simulink model "ES209A_CurrMeasCorrln"  (R2013b)
settings: Solver=FixedStepDiscrete  SolverMode=SingleTasking  StartTime=0.0  StopTime=1  FixedStep=0.000125  RelTol=1e-3
values from neighbouring files (symbols this model uses):
  CurrMeasCorrlnMaxErrCurr = DataDict.Calibration    [ES209A_CurrMeasCorrln_DataDict.m]
  CurrMeasCorrlnMaxStallCntr = DataDict.Calibration    [ES209A_CurrMeasCorrln_DataDict.m]
  CurrMeasCorrlnNtc0x04DFailStep = DataDict.Calibration    [ES209A_CurrMeasCorrln_DataDict.m]
  CurrMeasCorrlnNtc0x04DPassStep = DataDict.Calibration    [ES209A_CurrMeasCorrln_DataDict.m]
  CurrMeasCorrlnNtc0x04EFailStep = DataDict.Calibration    [ES209A_CurrMeasCorrln_DataDict.m]
  CurrMeasCorrlnNtc0x04EPassStep = DataDict.Calibration    [ES209A_CurrMeasCorrln_DataDict.m]
  ELECGLBPRM_IVTRCNT_CNT_U08 = DataDict.ConfigParam    [ES209A_CurrMeasCorrln_DataDict.m]
  FLTINJ_CURRMEASCORRLN_CURRMEASIDPTSIG = DataDict.Constant    [ES209A_CurrMeasCorrln_DataDict.m]
libraries: NxtrLim x2, simulink x1
(part 1 of 2)
settings Model: Creator=hzy4g9  LastModifiedBy=wzvp6q
settings SolverCC: AutoInsertRateTranBlk=on  InsertRTBMode=Always
settings DataIOCC: LimitDataPoints=off  SaveFormat=Structure  ReturnWorkspaceOutputs=on
settings OptimizationCC: BlockReduction=off  InlineParams=on  ZeroExternalMemoryAtStartup=off  ZeroInternalMemoryAtStartup=off  OptimizeModelRefInitCode=on  LifeSpan=1
settings DebuggingCC: SignalInfNanChecking=error  SignalRangeChecking=warning  UnderspecifiedInitializationDetection=Simplified  SolverPrmCheckMsg=error  InheritedTsInSrcMsg=error  DiscreteInheritContinuousMsg=error  SingleTaskRateTransMsg=error  TasksWithSamePriorityMsg=error  SigSpecEnsureSampleTimeMsg=error  CheckMatrixSingularityMsg=error  ParameterUnderflowMsg=error  ParameterPrecisionLossMsg=error  ParameterTunabilityLossMsg=error  FixptConstUnderflowMsg=warning  FixptConstOverflowMsg=warning  VectorMatrixConversionMsg=error  SignalLabelMismatchMsg=error  UnconnectedInputMsg=error  UnconnectedOutputMsg=error  UnconnectedLineMsg=error  SFcnCompatibilityMsg=error  UniqueDataStoreMsg=warning  BusObjectLabelMismatch=error  RootOutportRequireBusObject=error  AssertControl=DisableAll  ModelReferenceIOMsg=error  ModelReferenceVersionMismatchMessage=warning  ModelReferenceIOMismatchMessage=error  ModelReferenceCSMismatchMessage=warning  ModelReferenceDataLoggingMessage=error  StateNameClashWarn=warning  StrictBusMsg=ErrorOnBusTreatedAsVector  NonBusSignalsTreatedAsBus=error  SFUnexpectedBacktrackingDiag=error  SFInvalidInputDataAccessInChartInitDiag=error  SFNoUnconditionalDefaultTransitionDiag=error  SFTransitionOutsideNaturalParentDiag=error  SFUnconditionalTransitionShadowingDiag=error  SFUndirectedBroadcastEventsDiag=error
settings ModelReferenceCC: ModelReferenceNumInstancesAllowed=Single
settings RTWCC: SystemTargetFile=autosar.tlc  GenCodeOnly=on  TemplateMakefile=ert_default_tmf  Description=AUTOSAR  GenerateReport=on  ProcessScript=autosar_make_rtw_hook  LaunchReport=on
settings CodeAppCC: GenerateComments=off  IgnoreCustomStorageClasses=off  CustomSymbolStrType=$N$R$M  CustomSymbolStrBlkIO=$N$M  SimulinkBlockComments=off
settings STFCustomTargetCC: ParMdlRefBuildCompliant=on  CompOptLevelCompliant=on  IncludeMdlTerminateFcn=off  CombineOutputUpdateFcns=on  SuppressErrorStatus=on  ERTFirstTimeCompliant=on  ERTCustomFileBanners=on  SupportNonFinite=off  SupportComplex=off  SupportContinuousTime=off  SupportNonInlinedSFcns=off  MATLABClassNameForMDSCustomization=Simulink.SoftwareTarget.ERTCustomization  AutosarCompliant=on  GRTInterface=off  SystemTargetFile=autosar.tlc
settings ERTTargetCC: CodeReplacementLibrary=ANSI_C  ConcurrentExecutionCompliant=off  IncludeMdlTerminateFcn=off  SuppressErrorStatus=on  SupportNonFinite=off  SupportComplex=off  ModelStepFunctionPrototypeControlCompliant=off  CPPClassGenCompliant=off  AutosarCompliant=on  InlinedParameterPlacement=NonHierarchical  ERTCustomFileTemplate=example_file_process.tlc  EnableUserReplacementTypes=on

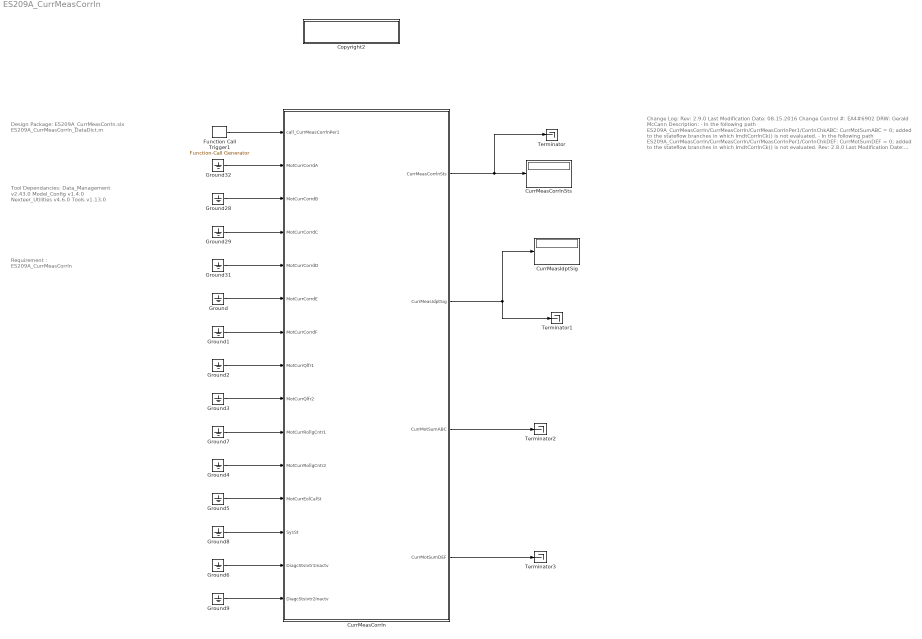
== system ES209A_CurrMeasCorrln ==
  note: Design Package:
      |
      | ES209A_CurrMeasCorrln.slx
      | ES209A_CurrMeasCorrln_DataDict.m
  note: Tool Dependancies:
      |
      | Data_Management v2.43.0
      | Model_Config v1.4.0
      | Nexteer_Utilities v4.6.0
      | Tools v1.13.0
  note: Requirement :
      |
      | ES209A_CurrMeasCorrln
  note: Change Log:
      |
      | Rev: 2.9.0
      | Last Modification Date: 08.15.2016
      | Change Control #: EA4#6902
      | DRW: Gerald McCann
      | Description:
      | - In the following path ES209A_CurrMeasCorrln/CurrMeasCorrln/CurrMeasCorrlnPer1/CorrlnChkABC:
      |    CurrMotSumABC = 0; added to the stateflow branches in which ImdtCorrlnCk() is not evaluated.
      | - In the following path ES209A_CurrMeasCorrln/CurrMeasCorrln/CurrMeasCorrlnPer1/CorrlnChkDEF:
      |    CurrMotSumDEF = 0; added to the stateflow branches in which ImdtCorrlnCk() is not evaluated.
      |
      | Rev: 2.8.0
      | Last Modification Date: 07.11.2016
      | Change Control #: EA4#6478
      | DRW: Gerald McCann
      | Description:
      | - In the following path, change the name of return value of ImdtCorrlnCk from CorrlnCk to ImdtCorrlnABC to match simulink block
      |    ES209A_CurrMeasCorrln/CurrMeasCorrln/CurrMeasCorrlnPer1/CorrlnChkABC
      | - In the following path, change the name of return value of ImdtCorrlnCk from CorrlnCk to ImdtCorrlnDEF to match simulink block
      |    ES209A_CurrMeasCorrln/CurrMeasCorrln/CurrMeasCorrlnPer1/CorrlnChkDEF
      | - In the following path, second condition [StallCntOutp >= kMaxStallCnt] changed to first condition.
      |    - ES209A_CurrMeasCorrln/CurrMeasCorrln/CurrMeasCorrlnPer1/Signal Availability/SigAvlChk1/SigAvlChkRev2
      | - Added return parameter CurrMotSum to ImdtCorrlnCk.  Source code unaffected as
      |    implementation already makes use of CurrMotSum.
      | - In stateflow CorrlnChkABC
      |    - Constant NTCNR_0X04D initial value changed to 77
      |    - Constant NTCNR_0X04D DataType changed to uint16
      | - In stateflow CorrlnChkDEF
      |    - Constant NTCNR_0X04E initial value changed to 78
      |    - Constant NTCNR_0X04E DataType changed to uint16
      | - Diagnostics warnings, Read Before Write, Write After Read and Write After Write has been
      |    changed to 'none' for the following blocks: NtcQlfr4D and NtcQlfr4E
      | - For simulation purposes only block ISO Fault Debounce Design stateflow has been modified
      |    to eliminate unconditional transitions
      | - Removed output port labels in the following paths due to signal label mismatch:
      |    - ES209A_CurrMeasCorrln/CurrMeasCorrln/CurrMeasCorrlnPer1/CorrlnChkABC/SetNtcSts/SetNtcSts/ISO Fault Debounce Design
      |    - ES209A_CurrMeasCorrln/CurrMeasCorrln/CurrMeasCorrlnPer1/CorrlnChkDEF/SetNtcSts/SetNtcSts/ISO Fault Debounce Design
      |
      | Rev: 2.7.0
      | Last Modification Date: 06.16.2016
      | Change Control #: EA4#6036
      | DRW: Raghavendran Mohan
      | Description:
      | - Added Fault Injection Mechanism for CurrMeasIdptSig
      |
      | Rev: 2.6.0
      | Last Modification Date: 04.22.2016
      | Change Control #: EA4#5281
      | DRW: Gerald McCann
      | Description:
      | - Signal Availability check is enabled only in enable/operate state.
      |
      | Rev: 2.5.0
      | Last Modification Date: 04.08.2016
      | Change Control #: EA4#5061
      | DRW: Praveen Devaraj(KPIT)
      | Description:
      | - Added two outputs CurrMotSumABC,CurrMotSumDEF and limiter added for these outputs.
      |
      | Rev: 2.4.0
      | Last Modification Date: 03.15.2016
      | Change Control #: Anomaly # EA4#2989     Comp   EA4#4533	     WCR # EA4#4747
      | DRW: N. Mahmud
      | Description:
      | - Fixed the datatype mismatch on CurrMeasCorrlnSts connection
      |
      | Rev: 2.3.0
      | Last Modification Date: 01.08.2016
      | Change Control #: EA4#2628	WCR # EA4#3283
      | DRW: N. Mahmud
      | Description:
      | - Requirement Linkage has been updated for the change described in the last version (Rev 2.2.0)
      |
      | Rev: 2.2.0
      | Last Modification Date: 12.07.2015
      | Change Control #: EA4#2628	WCR # EA4#2938
      | DRW: N. Mahmud
      | Description:
      | - Logic change in the number of independent signal  calculation for common mode failiure
      | - Change the kMaxStallCnt cal from 20 to 200 in the m file
      |
      | Rev: 2.1.0
      | Last Modification Date: 09.23.2015
      | Change Control #: WCR#1670
      | DRW: N. Mahmud
      | Description:
      | - Diagnostics has been disabled when gain/offset active: MotCurrEolCalSt is used to check that
      | - CurrMeasImdtCorrlnStsVldABC, CurrMeasLongTermCorrlnStsVldABC,
      |   CurrMeasImdtCorrlnStsVldDEF, CurrMeasLongTermCorrlnStsVldDEF are set to 1 as default.
      |
      | Rev: 1.0.0
      | Last Modification Date: 06.09.2015
      | Change Control #: ICR-
      | DRW: N. Mahmud
      | Description:
      | - Initial Release
      |
      | DRW: Nayeem Mahmud
      | Description:
      | ES209A Current Measurement Correlation
  Copyright2 : Subsystem  Description=|  mask(Copyright Information){none=on}
      | Copyright info block.                                               
      |                                                                     
      | Place copyright information at the top of every subsystem in design.
      mask prompts: none "No parameters"
      mask help: Place copyright information at the top of every subsystem in design.
      mask Display:
      | NxtrConf = 'Nexteer Confidential';
      | 
      | sys = bdroot; %handle for the current model ("system")
      | first = get_param(sys,'Created');
      | if(isempty(first))
      |     first = datestr(now,'yyyy');
      | else
      |     first = first(end-3:end);  %year is last four digits
      | end
      | 
      | last = get_param(sys,'LastModifiedDate');
      | if isempty(last)
      |     last = datestr(now,'yyyy');
      | else
      |     last = last(end-3:end);
      | end
      | 
      | if strcmp(first,last)
      |     fprintf('%s\nCopyright  %s Nexteer',NxtrConf,first);
      | else
      |     fprintf('%s\n%s%s-%s Nexteer',NxtrConf,char(169),first,last);
      | end
  CurrMeasCorrln : Subsystem  RequirementInfo={} %GIDa_ec0b3b79_5a07_49bd_97c9_8e172166434e
  CurrMeasCorrlnSts : Display
  CurrMeasIdptSig : Display
  Function Call Trigger1 : simulink/Ports & Subsystems/Function-Call Generator  RequirementInfo={} %GIDa_00b61420_5682_4f19_899b_6da543d44005  sample_time=0.000125  numberOfIterations=1
  Ground{,1..9,28..29,31..32} (14 alike) : Ground
  Terminator{,1..3} (4 alike) : Terminator
  wires:
  CurrMeasCorrln/1(CurrMeasCorrlnSts) -> Terminator/1, CurrMeasCorrlnSts/1
  CurrMeasCorrln/2(CurrMeasIdptSig) -> Terminator1/1, CurrMeasIdptSig/1
  Function Call Trigger1/1 -> CurrMeasCorrln/1(call_CurrMeasCorrlnPer1)
  Ground5/1 -> CurrMeasCorrln/12(MotCurrEolCalSt)
  Ground7/1 -> CurrMeasCorrln/10(MotCurrRollgCntr1)
  Ground28/1 -> CurrMeasCorrln/3(MotCurrCorrdB)
  Ground4/1 -> CurrMeasCorrln/11(MotCurrRollgCntr2)
  Ground9/1 -> CurrMeasCorrln/15(DiagcStsIvtr2Inactv)
  Ground6/1 -> CurrMeasCorrln/14(DiagcStsIvtr1Inactv)
  Ground31/1 -> CurrMeasCorrln/5(MotCurrCorrdD)
  Ground29/1 -> CurrMeasCorrln/4(MotCurrCorrdC)
  Ground2/1 -> CurrMeasCorrln/8(MotCurrQlfr1)
  Ground/1 -> CurrMeasCorrln/6(MotCurrCorrdE)
  Ground32/1 -> CurrMeasCorrln/2(MotCurrCorrdA)
  Ground8/1 -> CurrMeasCorrln/13(SysSt)
  Ground3/1 -> CurrMeasCorrln/9(MotCurrQlfr2)
  Ground1/1 -> CurrMeasCorrln/7(MotCurrCorrdF)
  CurrMeasCorrln/3(CurrMotSumABC) -> Terminator2/1
  CurrMeasCorrln/4(CurrMotSumDEF) -> Terminator3/1

== system ES209A_CurrMeasCorrln/Copyright2 ==

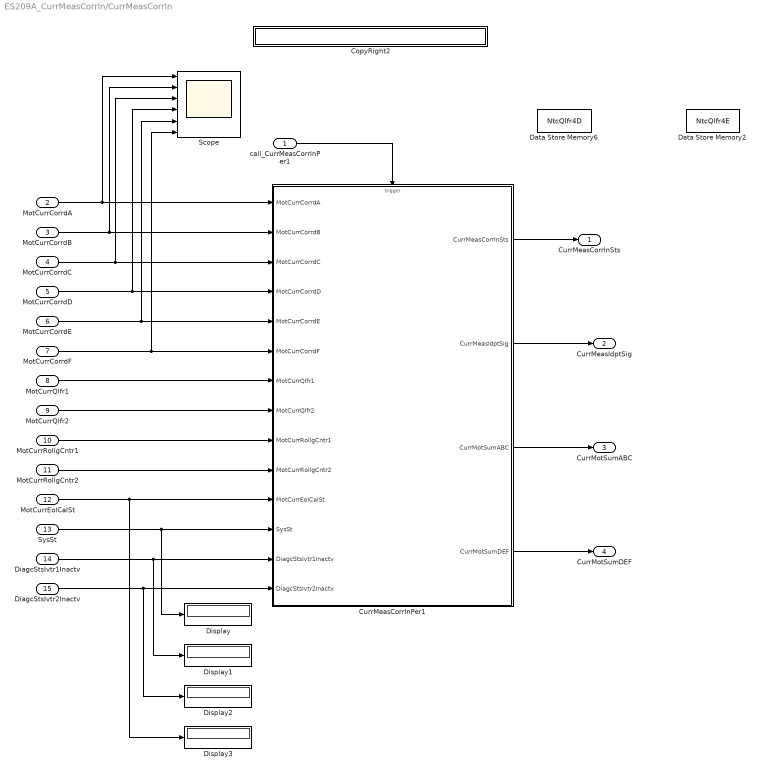
== system ES209A_CurrMeasCorrln/CurrMeasCorrln ==
  call_CurrMeasCorrlnPer1 : Inport
  MotCurrCorrdA : Inport  RequirementInfo={'linktype_rmi_doors' '0000c46e (/ESG Group/FDD Module Requirements/EA4 Specific/ES209A CurrMeasCorrln)' '#ES209A_104' 'true' 'REQ: ES209A_104' '' } %GIDa_0c74aa9f_9e88_4fad_92c6_c1c5b5def755  Port=2  OutDataTypeStr=single
  MotCurrCorrdB : Inport  RequirementInfo={'linktype_rmi_doors' '0000c46e (/ESG Group/FDD Module Requirements/EA4 Specific/ES209A CurrMeasCorrln)' '#ES209A_103' 'true' 'REQ: ES209A_103' '' } %GIDa_c4f83946_697c_4fbf_99fc_1a7b01ac928b  Port=3  OutDataTypeStr=single
  MotCurrCorrdC : Inport  RequirementInfo={'linktype_rmi_doors' '0000c46e (/ESG Group/FDD Module Requirements/EA4 Specific/ES209A CurrMeasCorrln)' '#ES209A_102' 'true' 'REQ: ES209A_102' '' } %GIDa_e8bdbe1c_0de3_460c_add6_42db4b0bf916  Port=4  OutDataTypeStr=single
  MotCurrCorrdD : Inport  RequirementInfo={'linktype_rmi_doors' '0000c46e (/ESG Group/FDD Module Requirements/EA4 Specific/ES209A CurrMeasCorrln)' '#ES209A_101' 'true' 'REQ: ES209A_101' '' } %GIDa_5fd63c82_c940_4205_a4b2_8a6f33b322f4  Port=5  OutDataTypeStr=single
  MotCurrCorrdE : Inport  RequirementInfo={'linktype_rmi_doors' '0000c46e (/ESG Group/FDD Module Requirements/EA4 Specific/ES209A CurrMeasCorrln)' '#ES209A_100' 'true' 'REQ: ES209A_100' '' } %GIDa_43c493df_4f0a_42bf_8466_dc5b3f8ce965  Port=6  OutDataTypeStr=single
  MotCurrCorrdF : Inport  RequirementInfo={'linktype_rmi_doors' '0000c46e (/ESG Group/FDD Module Requirements/EA4 Specific/ES209A CurrMeasCorrln)' '#ES209A_99' 'true' 'REQ: ES209A_99' '' } %GIDa_9f9bc708_ebce_4b8f_aa37_758e3dd2df64  Port=7  OutDataTypeStr=single
  MotCurrQlfr1 : Inport  RequirementInfo={'linktype_rmi_doors' '0000c46e (/ESG Group/FDD Module Requirements/EA4 Specific/ES209A CurrMeasCorrln)' '#ES209A_215' 'true' 'REQ: ES209A_215' '' } %GIDa_aa88c4e2_69a0_4fc7_a614_d2a8879a5609  Port=8
  MotCurrQlfr2 : Inport  RequirementInfo={'linktype_rmi_doors' '0000c46e (/ESG Group/FDD Module Requirements/EA4 Specific/ES209A CurrMeasCorrln)' '#ES209A_214' 'true' 'REQ: ES209A_214' '' } %GIDa_eed2eea5_fe21_4beb_a317_55bd282b43d2  Port=9
  MotCurrRollgCntr1 : Inport  RequirementInfo={'linktype_rmi_doors' '0000c46e (/ESG Group/FDD Module Requirements/EA4 Specific/ES209A CurrMeasCorrln)' '#ES209A_213' 'true' 'REQ: ES209A_213' '' } %GIDa_0df31c93_de9f_4bc8_bb2d_b19ad16d92b3  Port=10
  MotCurrRollgCntr2 : Inport  RequirementInfo={'linktype_rmi_doors' '0000c46e (/ESG Group/FDD Module Requirements/EA4 Specific/ES209A CurrMeasCorrln)' '#ES209A_212' 'true' 'REQ: ES209A_212' '' } %GIDa_a808d1c9_e453_4f42_bcf3_8307b2c8619b  Port=11
  MotCurrEolCalSt : Inport  RequirementInfo={} %GIDa_abcbe149_f782_4267_9a45_157caba417ed  Port=12
  SysSt : Inport  RequirementInfo={} %GIDa_8538c24b_5f6a_4d2a_9d09_038d40d09e05  Port=13  OutDataTypeStr=uint8
  DiagcStsIvtr1Inactv : Inport  RequirementInfo={} %GIDa_38774f0c_8ba6_46af_9c68_e8c1be2e73a7  Port=14  OutDataTypeStr=boolean
  DiagcStsIvtr2Inactv : Inport  RequirementInfo={} %GIDa_811cc2e1_8a27_4ac8_82c1_1322cbb91599  Port=15  OutDataTypeStr=boolean
  CopyRight2 : Subsystem  Description=|  mask(Copyright Information){none=on}
      | Copyright info block.                                               
      |                                                                     
      | Place copyright information at the top of every subsystem in design.
      mask prompts: none "No parameters"
      mask help: Place copyright information at the top of every subsystem in design.
      mask Display:
      | NxtrConf = 'Nexteer Confidential';
      | 
      | sys = bdroot; %handle for the current model ("system")
      | first = get_param(sys,'Created');
      | first = first(end-3:end);  %year is last four digits
      | 
      | last = get_param(sys,'LastModifiedDate');
      | if isempty(last)
      |     last = datestr(now,'yyyy');
      | else
      |     last = last(end-3:end);
      | end
      | 
      | if strcmp(first,last)
      |     fprintf('%s -- Copyright %s Nexteer',NxtrConf,first)
      | else
      |     fprintf('%s -- %s%s- %s Nexteer',NxtrConf,char(169),first,last)
      | end
  CurrMeasCorrlnPer1 : Subsystem  RequirementInfo={'linktype_rmi_doors' '0000c46e (/ESG Group/FDD Module Requirements/EA4 Specific/ES209A CurrMeasCorrln)' '#ES209A_262' 'true' 'REQ: ES209A_262' '' } %GIDa_55579703_5885_40a5_a6ff_7209441b4d74  TreatAsAtomicUnit=on
  Data Store Memory2 : DataStoreMemory  DataStoreName=NtcQlfr4E  OutDataTypeStr=uint8
      settings: AttributesFormatString=|
      | Simulation Purpose Only.
      | Do Not Code this block
      | Diagnostic Manager Owns this requirement
  Data Store Memory6 : DataStoreMemory  DataStoreName=NtcQlfr4D  OutDataTypeStr=uint8
      settings: AttributesFormatString=|
      | Simulation Purpose Only.
      | Do Not Code this block
      | Diagnostic Manager Owns this requirement
  Display{,1..3} (4 alike) : Display
  Scope : Scope  NumInputPorts=6
      settings: YMin=-30~-30~-5~-5~-5~-5  YMax=30~25~5~5~5~5  SaveName=ScopeData2
  CurrMeasCorrlnSts : Outport  RequirementInfo={'linktype_rmi_doors' '0000c46e (/ESG Group/FDD Module Requirements/EA4 Specific/ES209A CurrMeasCorrln)' '#ES209A_205' 'true' 'REQ: ES209A_205' '' } %GIDa_1cc70fdd_56e1_4fc7_8a0b_3b5472613135
  CurrMeasIdptSig : Outport  RequirementInfo={'linktype_rmi_doors' '0000c46e (/ESG Group/FDD Module Requirements/EA4 Specific/ES209A CurrMeasCorrln)' '#ES209A_216' 'true' 'REQ: ES209A_216' '' } %GIDa_d8a59612_7cd1_4e21_946e_1ecb99779eae  Port=2
  CurrMotSumABC : Outport  RequirementInfo={'linktype_rmi_doors' '0000c46e (/ESG Group/FDD Module Requirements/EA4 Specific/ES209A_CurrMeasCorrln)' '#ES209A_276' 'true' 'REQ: ES209A_276' '' } %GIDa_6a109cf6_d31d_4752_8888_2bcd8313dc3b  Port=3
  CurrMotSumDEF : Outport  RequirementInfo={'linktype_rmi_doors' '0000c46e (/ESG Group/FDD Module Requirements/EA4 Specific/ES209A_CurrMeasCorrln)' '#ES209A_277' 'true' 'REQ: ES209A_277' '' } %GIDa_ea0a91c7_9f07_4e8d_b88b_4e34ddd11616  Port=4
  wires:
  call_CurrMeasCorrlnPer1/1 -> CurrMeasCorrlnPer1/Trigger
  MotCurrCorrdC/1 -> Scope/3, CurrMeasCorrlnPer1/3(MotCurrCorrdC)
  MotCurrCorrdA/1 -> Scope/1, CurrMeasCorrlnPer1/1(MotCurrCorrdA)
  MotCurrCorrdD/1 -> Scope/4, CurrMeasCorrlnPer1/4(MotCurrCorrdD)
  MotCurrQlfr1/1 -> CurrMeasCorrlnPer1/7(MotCurrQlfr1)
  MotCurrCorrdF/1 -> Scope/6, CurrMeasCorrlnPer1/6(MotCurrCorrdF)
  MotCurrCorrdB/1 -> Scope/2, CurrMeasCorrlnPer1/2(MotCurrCorrdB)
  MotCurrQlfr2/1 -> CurrMeasCorrlnPer1/8(MotCurrQlfr2)
  MotCurrRollgCntr1/1 -> CurrMeasCorrlnPer1/9(MotCurrRollgCntr1)
  MotCurrRollgCntr2/1 -> CurrMeasCorrlnPer1/10(MotCurrRollgCntr2)
  MotCurrCorrdE/1 -> Scope/5, CurrMeasCorrlnPer1/5(MotCurrCorrdE)
  CurrMeasCorrlnPer1/1(CurrMeasCorrlnSts) -> CurrMeasCorrlnSts/1
  CurrMeasCorrlnPer1/2(CurrMeasIdptSig) -> CurrMeasIdptSig/1
  MotCurrEolCalSt/1 -> Display3/1, CurrMeasCorrlnPer1/11(MotCurrEolCalSt)
  SysSt/1 -> Display/1, CurrMeasCorrlnPer1/12(SysSt)
  DiagcStsIvtr1Inactv/1 -> Display1/1, CurrMeasCorrlnPer1/13(DiagcStsIvtr1Inactv)
  DiagcStsIvtr2Inactv/1 -> Display2/1, CurrMeasCorrlnPer1/14(DiagcStsIvtr2Inactv)
  CurrMeasCorrlnPer1/3(CurrMotSumABC) -> CurrMotSumABC/1
  CurrMeasCorrlnPer1/4(CurrMotSumDEF) -> CurrMotSumDEF/1

== system ES209A_CurrMeasCorrln/CurrMeasCorrln/CopyRight2 ==

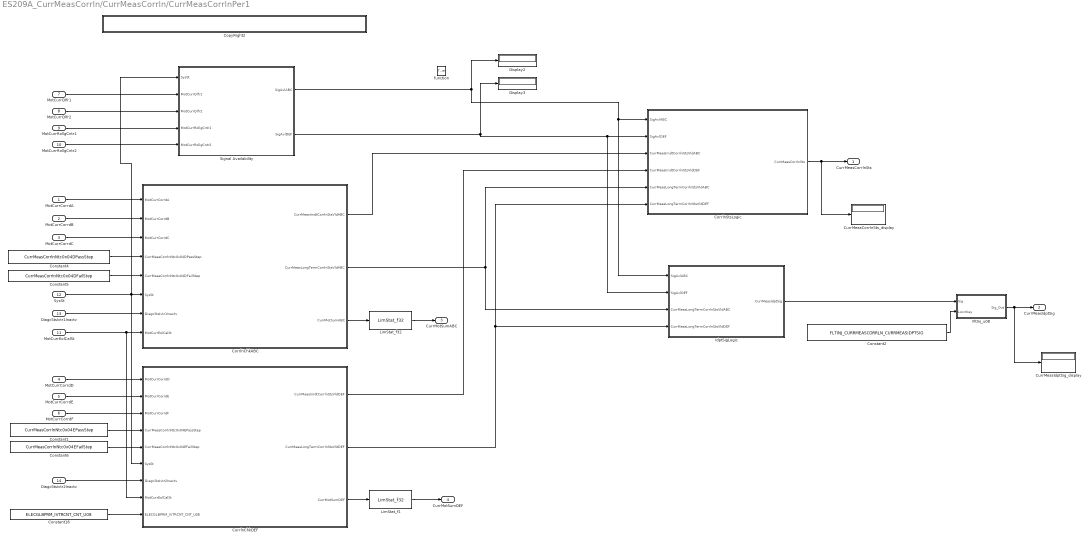
== system ES209A_CurrMeasCorrln/CurrMeasCorrln/CurrMeasCorrlnPer1 ==
  MotCurrCorrdA : Inport  RequirementInfo={} %GIDa_1b4be831_2b7f_4bad_8ca7_c41d6d58feee
  MotCurrCorrdB : Inport  RequirementInfo={} %GIDa_500faeb4_9506_45cf_9bc9_0622a43ff9e4  Port=2
  MotCurrCorrdC : Inport  RequirementInfo={} %GIDa_bdd58e2d_11b0_4592_a6cb_cf558d278bca  Port=3
  MotCurrCorrdD : Inport  RequirementInfo={} %GIDa_1787db15_a767_43f2_bc85_acb71f8d69c6  Port=4
  MotCurrCorrdE : Inport  RequirementInfo={} %GIDa_b914ba1e_8e7d_4f95_9ec4_a4f9530234f8  Port=5
  MotCurrCorrdF : Inport  RequirementInfo={} %GIDa_90fedd66_ffe2_4248_b2d7_fc88368a78d6  Port=6
  MotCurrQlfr1 : Inport  RequirementInfo={} %GIDa_549edda9_9c07_47e0_960b_2f7219c5afa3  Port=7
  MotCurrQlfr2 : Inport  RequirementInfo={} %GIDa_6f0dc6ab_4498_4871_aa7d_039a645c93f3  Port=8
  MotCurrRollgCntr1 : Inport  RequirementInfo={} %GIDa_941568a4_4b86_4eee_9c4b_01a9e8a0d271  Port=9
  MotCurrRollgCntr2 : Inport  RequirementInfo={} %GIDa_6bb84625_6e4a_46ad_a031_3a9a545a3e69  Port=10
  MotCurrEolCalSt : Inport  RequirementInfo={'linktype_rmi_doors' '0000c46e (/ESG Group/FDD Module Requirements/EA4 Specific/ES209A CurrMeasCorrln)' '#ES209A_263' 'true' 'REQ: ES209A_263' '' ; 'linktype_rmi_doors' '0000c46e (/ESG Group/FDD Module Requirements/EA4 Specific/ES209A CurrMeasCorrln)' '#ES209A_264' 'true' 'REQ: ES209A_264' '' ; 'linktype_rmi_doors' '0000c46e (/ESG Group/FDD Module Requirements/EA4 Specific/ES209A CurrMeasCorrln)' '#ES209A_263' 'true' 'REQ: ES209A_263' '' } %GIDa_c49b2222_d3c8_435a_aa49_2a5d2eee96f8  Port=11
  SysSt : Inport  RequirementInfo={'linktype_rmi_doors' '0000c46e (/ESG Group/FDD Module Requirements/EA4 Specific/ES209A CurrMeasCorrln)' '#ES209A_263' 'true' 'REQ: ES209A_263' '' ; 'linktype_rmi_doors' '0000c46e (/ESG Group/FDD Module Requirements/EA4 Specific/ES209A CurrMeasCorrln)' '#ES209A_264' 'true' 'REQ: ES209A_264' '' ; 'linktype_rmi_doors' '0000c46e (/ESG Group/FDD Module Requirements/EA4 Specific/ES209A CurrMeasCorrln)' '#ES209A_263' 'true' 'REQ: ES209A_263' '' } %GIDa_7eb989da_9939_43d3_b23d_4ca6ddd74654  Port=12  OutDataTypeStr=uint8
  DiagcStsIvtr1Inactv : Inport  RequirementInfo={'linktype_rmi_doors' '0000c46e (/ESG Group/FDD Module Requirements/EA4 Specific/ES209A CurrMeasCorrln)' '#ES209A_263' 'true' 'REQ: ES209A_263' '' ; 'linktype_rmi_doors' '0000c46e (/ESG Group/FDD Module Requirements/EA4 Specific/ES209A CurrMeasCorrln)' '#ES209A_263' 'true' 'REQ: ES209A_263' '' ; 'linktype_rmi_doors' '0000c46e (/ESG Group/FDD Module Requirements/EA4 Specific/ES209A CurrMeasCorrln)' '#ES209A_265' 'true' 'REQ: ES209A_265' '' } %GIDa_52cd4757_636a_4123_80e9_de329e501eb0  Port=13
  DiagcStsIvtr2Inactv : Inport  RequirementInfo={'linktype_rmi_doors' '0000c46e (/ESG Group/FDD Module Requirements/EA4 Specific/ES209A CurrMeasCorrln)' '#ES209A_264' 'true' 'REQ: ES209A_264' '' ; 'linktype_rmi_doors' '0000c46e (/ESG Group/FDD Module Requirements/EA4 Specific/ES209A CurrMeasCorrln)' '#ES209A_265' 'true' 'REQ: ES209A_265' '' } %GIDa_ae52e87f_c4e9_4b70_9292_5a6f0defc3c4  Port=14
  function : TriggerPort  TriggerType=function-call
  Constant1 : Constant  Value=CurrMeasCorrlnNtc0x04EPassStep
  Constant18 : Constant  RequirementInfo={'linktype_rmi_doors' '0000c46e (/ESG Group/FDD Module Requirements/EA4 Specific/ES209A CurrMeasCorrln)' '#ES209A_264' 'true' 'REQ: ES209A_264' '' } %GIDa_30da442b_a6bf_42bc_be81_91df8133d060  Value=ELECGLBPRM_IVTRCNT_CNT_U08
  Constant2 : Constant  Value=FLTINJ_CURRMEASCORRLN_CURRMEASIDPTSIG
  Constant4 : Constant  Value=CurrMeasCorrlnNtc0x04DPassStep
  Constant5 : Constant  Value=CurrMeasCorrlnNtc0x04DFailStep
  Constant6 : Constant  Value=CurrMeasCorrlnNtc0x04EFailStep
  CopyRight2 : Subsystem  Description=|  mask(Copyright Information){none=on}
      | Copyright info block.                                               
      |                                                                     
      | Place copyright information at the top of every subsystem in design.
      mask prompts: none "No parameters"
      mask help: Place copyright information at the top of every subsystem in design.
      mask Display:
      | NxtrConf = 'Nexteer Confidential';
      | 
      | sys = bdroot; %handle for the current model ("system")
      | first = get_param(sys,'Created');
      | first = first(end-3:end);  %year is last four digits
      | 
      | last = get_param(sys,'LastModifiedDate');
      | if isempty(last)
      |     last = datestr(now,'yyyy');
      | else
      |     last = last(end-3:end);
      | end
      | 
      | if strcmp(first,last)
      |     fprintf('%s -- Copyright %s Nexteer',NxtrConf,first)
      | else
      |     fprintf('%s -- %s%s- %s Nexteer',NxtrConf,char(169),first,last)
      | end
  CorrlnChkABC : Stateflow chart  TreatAsAtomicUnit=on
  CorrlnChkDEF : Stateflow chart  TreatAsAtomicUnit=on
  CorrlnStsLogic : Subsystem  RequirementInfo={} %GIDa_a00f341f_7944_4604_9319_bb050268a085
  CurrMeasCorrlnSts_display : Display
  CurrMeasIdptSig_display : Display
  Display2 : Display
  Display3 : Display
  FltInj_u08 : Subsystem  RequirementInfo={'linktype_rmi_doors' '0000c46e (/ESG Group/FDD Module Requirements/EA4 Specific/ES209A_CurrMeasCorrln)' '#ES209A_280' 'true' 'REQ: ES209A_280' '' } %GIDa_04468b6b_fc20_408a_acd8_ab774034357d  TreatAsAtomicUnit=on  VariantControl=FLTINJENA ~= STD_ON  mask(Fault_Injection){}
      mask help: Simulation mode is just a pass-thru.
  IdptSigLogic : Subsystem  RequirementInfo={} %GIDa_ea49a6a8_9dd9_4522_a425_2915623b798a
  LimStat_f1 : NxtrLim/LimStat_f32  LoLim=CurrMotSumDEF.EngMin  HiLim=CurrMotSumDEF.EngMax
      settings: AttributesFormatString=|
      | Low Limit: %<LoLim>
      | High Limit:%<HiLim>
  LimStat_f32 : NxtrLim/LimStat_f32  LoLim=CurrMotSumABC.EngMin  HiLim=CurrMotSumABC.EngMax
      settings: AttributesFormatString=|
      | Low Limit: %<LoLim>
      | High Limit:%<HiLim>
  Signal Availability : Subsystem  RequirementInfo={} %GIDa_b157c1ee_10a9_448e_9e7d_b9c83f2081ec
  CurrMeasCorrlnSts : Outport  RequirementInfo={} %GIDa_7d108d83_7d1e_4d9a_a3d7_d8c403dededd
  CurrMeasIdptSig : Outport  RequirementInfo={} %GIDa_f7dae694_b925_4279_806a_2573b5172d71  Port=2
  CurrMotSumABC : Outport  Port=3
  CurrMotSumDEF : Outport  Port=4
  wires:
  MotCurrCorrdB/1 -> CorrlnChkABC/2(MotCurrCorrdB)
  MotCurrCorrdA/1 -> CorrlnChkABC/1(MotCurrCorrdA)
  Signal Availability/2(SigAvlDEF) -> IdptSigLogic/2(SigAvlDEF), CorrlnStsLogic/2(SigAvlDEF), Display3/1
  MotCurrCorrdC/1 -> CorrlnChkABC/3(MotCurrCorrdC)
  CorrlnChkABC/2(CurrMeasLongTermCorrlnStsVldABC) -> IdptSigLogic/3(CurrMeasLongTermCorrlnStsVldABC), CorrlnStsLogic/5(CurrMeasLongTermCorrlnStsVldABC)
  Constant4/1 -> CorrlnChkABC/4(CurrMeasCorrlnNtc0x04DPassStep)
  Constant5/1 -> CorrlnChkABC/5(CurrMeasCorrlnNtc0x04DFailStep)
  Constant1/1 -> CorrlnChkDEF/4(CurrMeasCorrlnNtc0x04EPassStep)
  Constant6/1 -> CorrlnChkDEF/5(CurrMeasCorrlnNtc0x04EFailStep)
  MotCurrCorrdD/1 -> CorrlnChkDEF/1(MotCurrCorrdD)
  MotCurrCorrdE/1 -> CorrlnChkDEF/2(MotCurrCorrdE)
  MotCurrCorrdF/1 -> CorrlnChkDEF/3(MotCurrCorrdF)
  DiagcStsIvtr2Inactv/1 -> CorrlnChkDEF/7(DiagcStsIvtr2Inactv)
  Constant18/1 -> CorrlnChkDEF/9(ELECGLBPRM_IVTRCNT_CNT_U08)
  SysSt/1 -> CorrlnChkDEF/6(SysSt), Signal Availability/1(SysSt), CorrlnChkABC/6(SysSt)
  DiagcStsIvtr1Inactv/1 -> CorrlnChkABC/7(DiagcStsIvtr1Inactv)
  MotCurrEolCalSt/1 -> CorrlnChkDEF/8(MotCurrEolCalSt), CorrlnChkABC/8(MotCurrEolCalSt)
  IdptSigLogic/1(CurrMeasIdptSig) -> FltInj_u08/1(Sig)
  CorrlnStsLogic/1(CurrMeasCorrlnSts) -> CurrMeasCorrlnSts_display/1, CurrMeasCorrlnSts/1
  Signal Availability/1(SigAvlABC) -> IdptSigLogic/1(SigAvlABC), CorrlnStsLogic/1(SigAvlABC), Display2/1
  CorrlnChkABC/1(CurrMeasImdtCorrlnStsVldABC) -> CorrlnStsLogic/3(CurrMeasImdtCorrlnStsVldABC)
  CorrlnChkDEF/1(CurrMeasImdtCorrlnStsVldDEF) -> CorrlnStsLogic/4(CurrMeasImdtCorrlnStsVldDEF)
  CorrlnChkDEF/2(CurrMeasLongTermCorrlnStsVldDEF) -> IdptSigLogic/4(CurrMeasLongTermCorrlnStsVldDEF), CorrlnStsLogic/6(CurrMeasLongTermCorrlnStsVldDEF)
  CorrlnChkABC/3(CurrMotSumABC) -> LimStat_f32/1
  CorrlnChkDEF/3(CurrMotSumDEF) -> LimStat_f1/1
  LimStat_f32/1 -> CurrMotSumABC/1
  LimStat_f1/1 -> CurrMotSumDEF/1
  MotCurrRollgCntr2/1 -> Signal Availability/5(MotCurrRollgCntr2)
  MotCurrRollgCntr1/1 -> Signal Availability/4(MotCurrRollgCntr1)
  MotCurrQlfr2/1 -> Signal Availability/3(MotCurrQlfr2)
  MotCurrQlfr1/1 -> Signal Availability/2(MotCurrQlfr1)
  FltInj_u08/1(Sig_Out) -> CurrMeasIdptSig_display/1, CurrMeasIdptSig/1
  Constant2/1 -> FltInj_u08/2("LocnKey  ")

== system ES209A_CurrMeasCorrln/CurrMeasCorrln/CurrMeasCorrlnPer1/CopyRight2 ==

== system ES209A_CurrMeasCorrln/CurrMeasCorrln/CurrMeasCorrlnPer1/CorrlnChkABC/GetNtcQlfrSts ==
  NtcNr : Inport
  f : TriggerPort  TriggerType=function-call
      settings: CopyFcn=Stateflow.SLINSF.SimulinkMan.removeBlockPreDeleteFcn  PreDeleteFcn=Stateflow.SLINSF.SimulinkMan.unsafePredeleteFcn
  CopyRight2 : Subsystem  Description=|  mask(Copyright Information){none=on}
      | Copyright info block.                                               
      |                                                                     
      | Place copyright information at the top of every subsystem in design.
      mask prompts: none "No parameters"
      mask help: Place copyright information at the top of every subsystem in design.
      mask Display:
      | NxtrConf = 'Nexteer Confidential';
      | 
      | sys = bdroot; %handle for the current model ("system")
      | first = get_param(sys,'Created');
      | first = first(end-3:end);  %year is last four digits
      | 
      | last = get_param(sys,'LastModifiedDate');
      | if isempty(last)
      |     last = datestr(now,'yyyy');
      | else
      |     last = last(end-3:end);
      | end
      | 
      | if strcmp(first,last)
      |     fprintf('%s -- Copyright %s Nexteer',NxtrConf,first)
      | else
      |     fprintf('%s -- %s%s- %s Nexteer',NxtrConf,char(169),first,last)
      | end
  Data Store Read1 : DataStoreRead  DataStoreName=NtcQlfr4D
  Terminator : Terminator
  NtcQlfr1 : Outport
  wires:
  NtcNr/1 -> Terminator/1
  Data Store Read1/1 -> NtcQlfr1/1

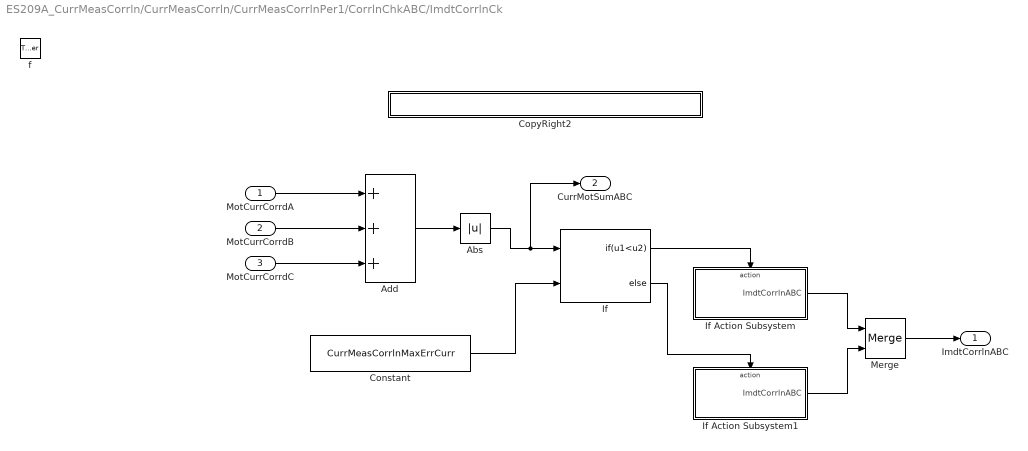
== system ES209A_CurrMeasCorrln/CurrMeasCorrln/CurrMeasCorrlnPer1/CorrlnChkABC/ImdtCorrlnCk ==
  MotCurrCorrdA : Inport  RequirementInfo={} %GIDa_0a2222ff_a94a_4249_a1bf_f32c3e06640e  OutDataTypeStr=double
  MotCurrCorrdB : Inport  RequirementInfo={} %GIDa_13b1c70b_2c56_462b_91dc_b07ad324a1f1  Port=2  OutDataTypeStr=double
  MotCurrCorrdC : Inport  RequirementInfo={} %GIDa_5c5b0a53_7fb0_4181_97a2_64d229646692  Port=3  OutDataTypeStr=double
  f : TriggerPort  TriggerType=function-call
      settings: CopyFcn=Stateflow.SLINSF.SimulinkMan.removeBlockPreDeleteFcn  PreDeleteFcn=Stateflow.SLINSF.SimulinkMan.unsafePredeleteFcn
  Abs : Abs  RequirementInfo={'linktype_rmi_doors' '0000c46e (/ESG Group/FDD Module Requirements/EA4 Specific/ES209A_CurrMeasCorrln)' '#ES209A_278' 'true' 'REQ: ES209A_278' '' } %GIDa_dda1e4f5_4799_45dc_b8fb_bab1482c5097
  Add : Sum  Inputs=+++
  Constant : Constant  Value=CurrMeasCorrlnMaxErrCurr  OutDataTypeStr=double
  CopyRight2 : Subsystem  Description=|  mask(Copyright Information){none=on}
      | Copyright info block.                                               
      |                                                                     
      | Place copyright information at the top of every subsystem in design.
      mask prompts: none "No parameters"
      mask help: Place copyright information at the top of every subsystem in design.
      mask Display:
      | NxtrConf = 'Nexteer Confidential';
      | 
      | sys = bdroot; %handle for the current model ("system")
      | first = get_param(sys,'Created');
      | first = first(end-3:end);  %year is last four digits
      | 
      | last = get_param(sys,'LastModifiedDate');
      | if isempty(last)
      |     last = datestr(now,'yyyy');
      | else
      |     last = last(end-3:end);
      | end
      | 
      | if strcmp(first,last)
      |     fprintf('%s -- Copyright %s Nexteer',NxtrConf,first)
      | else
      |     fprintf('%s -- %s%s- %s Nexteer',NxtrConf,char(169),first,last)
      | end
  If : If  RequirementInfo={'linktype_rmi_doors' '0000c46e (/ESG Group/FDD Module Requirements/EA4 Specific/ES209A CurrMeasCorrln)' '#ES209A_181' 'true' 'REQ: ES209A_181' '' ; 'linktype_rmi_doors' '0000c46e (/ESG Group/FDD Module Requirements/EA4 Specific/ES209A CurrMeasCorrln)' '#ES209A_249' 'true' 'REQ: ES209A_249' '' } %GIDa_87ba24c9_1ad1_422d_b8ed_ec7d69e4ed32  NumInputs=2  IfExpression=u1<u2
  If Action Subsystem : Subsystem  RequirementInfo={'linktype_rmi_doors' '0000c46e (/ESG Group/FDD Module Requirements/EA4 Specific/ES209A CurrMeasCorrln)' '#ES209A_249' 'true' 'REQ: ES209A_249' '' } %GIDa_04403ac0_7c86_42b2_ab61_c6af4afe39ec  TreatAsAtomicUnit=on
  If Action Subsystem1 : Subsystem  RequirementInfo={'linktype_rmi_doors' '0000c46e (/ESG Group/FDD Module Requirements/EA4 Specific/ES209A CurrMeasCorrln)' '#ES209A_181' 'true' 'REQ: ES209A_181' '' } %GIDa_2eb5824b_62d5_4f39_b24a_739b4084d937  TreatAsAtomicUnit=on
  Merge : Merge
  ImdtCorrlnABC : Outport
  CurrMotSumABC : Outport  Port=2
  wires:
  If/1 -> If Action Subsystem/Action
  MotCurrCorrdA/1 -> Add/1
  MotCurrCorrdC/1 -> Add/3
  MotCurrCorrdB/1 -> Add/2
  If/2 -> If Action Subsystem1/Action
  If Action Subsystem/1(ImdtCorrlnABC) -> Merge/1
  If Action Subsystem1/1(ImdtCorrlnABC) -> Merge/2
  Merge/1 -> ImdtCorrlnABC/1
  Add/1 -> Abs/1
  Constant/1 -> If/2
  Abs/1 -> CurrMotSumABC/1, If/1

== system ES209A_CurrMeasCorrln/CurrMeasCorrln/CurrMeasCorrlnPer1/CorrlnChkABC/SetNtcSts ==
  NTCNr : Inport
  ParamBit : Inport  Port=2
  NTCSts : Inport  Port=3
  NTCDebStep : Inport  Port=4
  f : TriggerPort  TriggerType=function-call
      settings: CopyFcn=Stateflow.SLINSF.SimulinkMan.removeBlockPreDeleteFcn  PreDeleteFcn=Stateflow.SLINSF.SimulinkMan.unsafePredeleteFcn
  CopyRight2 : Subsystem  Description=|  mask(Copyright Information){none=on}
      | Copyright info block.                                               
      |                                                                     
      | Place copyright information at the top of every subsystem in design.
      mask prompts: none "No parameters"
      mask help: Place copyright information at the top of every subsystem in design.
      mask Display:
      | NxtrConf = 'Nexteer Confidential';
      | 
      | sys = bdroot; %handle for the current model ("system")
      | first = get_param(sys,'Created');
      | first = first(end-3:end);  %year is last four digits
      | 
      | last = get_param(sys,'LastModifiedDate');
      | if isempty(last)
      |     last = datestr(now,'yyyy');
      | else
      |     last = last(end-3:end);
      | end
      | 
      | if strcmp(first,last)
      |     fprintf('%s -- Copyright %s Nexteer',NxtrConf,first)
      | else
      |     fprintf('%s -- %s%s- %s Nexteer',NxtrConf,char(169),first,last)
      | end
  Ground : Ground
  SetNtcSts : Subsystem  RequirementInfo={} %GIDa_994e7abf_9850_4f4e_86fd_7c163c9d2acc  TreatAsAtomicUnit=on
      settings: RTWSystemCode=Inline
  CurrMeasCorrlnNtcSet : Outport
  wires:
  Ground/1 -> CurrMeasCorrlnNtcSet/1
  NTCDebStep/1 -> SetNtcSts/4(DebStep)
  NTCSts/1 -> SetNtcSts/3(NtcSts)
  ParamBit/1 -> SetNtcSts/2(NtcStInfo)
  NTCNr/1 -> SetNtcSts/1(NtcNr)

== system ES209A_CurrMeasCorrln/CurrMeasCorrln/CurrMeasCorrlnPer1/CorrlnChkDEF/GetNtcQlfrSts ==
  NtcNr : Inport
  f : TriggerPort  TriggerType=function-call
      settings: CopyFcn=Stateflow.SLINSF.SimulinkMan.removeBlockPreDeleteFcn  PreDeleteFcn=Stateflow.SLINSF.SimulinkMan.unsafePredeleteFcn
  CopyRight2 : Subsystem  Description=|  mask(Copyright Information){none=on}
      | Copyright info block.                                               
      |                                                                     
      | Place copyright information at the top of every subsystem in design.
      mask prompts: none "No parameters"
      mask help: Place copyright information at the top of every subsystem in design.
      mask Display:
      | NxtrConf = 'Nexteer Confidential';
      | 
      | sys = bdroot; %handle for the current model ("system")
      | first = get_param(sys,'Created');
      | first = first(end-3:end);  %year is last four digits
      | 
      | last = get_param(sys,'LastModifiedDate');
      | if isempty(last)
      |     last = datestr(now,'yyyy');
      | else
      |     last = last(end-3:end);
      | end
      | 
      | if strcmp(first,last)
      |     fprintf('%s -- Copyright %s Nexteer',NxtrConf,first)
      | else
      |     fprintf('%s -- %s%s- %s Nexteer',NxtrConf,char(169),first,last)
      | end
  Data Store Read1 : DataStoreRead  DataStoreName=NtcQlfr4E
  Terminator : Terminator
  NtcQlfr1 : Outport
  wires:
  NtcNr/1 -> Terminator/1
  Data Store Read1/1 -> NtcQlfr1/1

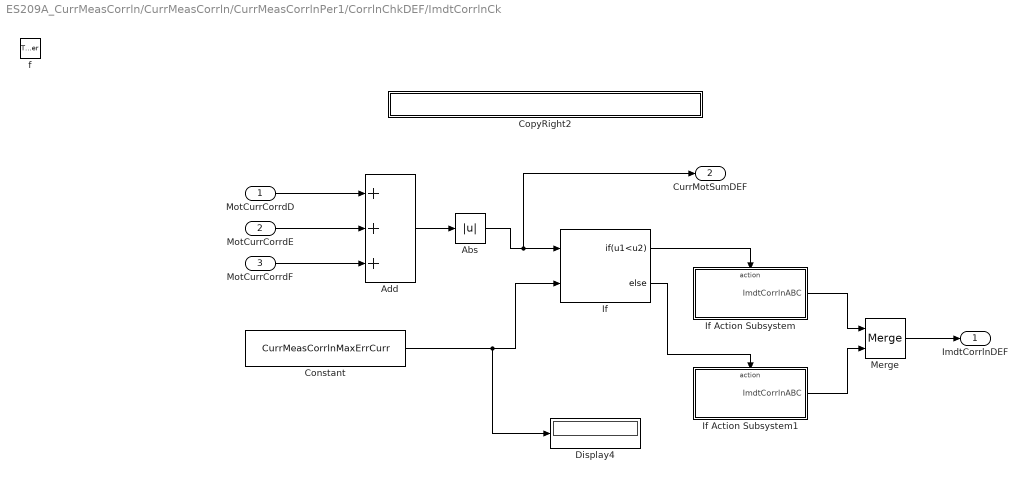
== system ES209A_CurrMeasCorrln/CurrMeasCorrln/CurrMeasCorrlnPer1/CorrlnChkDEF/ImdtCorrlnCk ==
  MotCurrCorrdD : Inport  RequirementInfo={} %GIDa_1ea4fc3e_97a5_4f6e_ace9_314441d11092  OutDataTypeStr=double
  MotCurrCorrdE : Inport  RequirementInfo={} %GIDa_e34f3d26_d1a6_489f_bea9_b26f91091d01  Port=2  OutDataTypeStr=double
  MotCurrCorrdF : Inport  RequirementInfo={} %GIDa_59ecd8a4_f9e4_49dc_abf2_186257832f32  Port=3  OutDataTypeStr=double
  f : TriggerPort  TriggerType=function-call
      settings: CopyFcn=Stateflow.SLINSF.SimulinkMan.removeBlockPreDeleteFcn  PreDeleteFcn=Stateflow.SLINSF.SimulinkMan.unsafePredeleteFcn
  Abs : Abs  RequirementInfo={'linktype_rmi_doors' '0000c46e (/ESG Group/FDD Module Requirements/EA4 Specific/ES209A_CurrMeasCorrln)' '#ES209A_279' 'true' 'REQ: ES209A_279' '' } %GIDa_76e9fdc7_c81c_48b1_b77d_b74f2a056a1c
  Add : Sum  Inputs=+++
  Constant : Constant  Value=CurrMeasCorrlnMaxErrCurr  OutDataTypeStr=double
  CopyRight2 : Subsystem  Description=|  mask(Copyright Information){none=on}
      | Copyright info block.                                               
      |                                                                     
      | Place copyright information at the top of every subsystem in design.
      mask prompts: none "No parameters"
      mask help: Place copyright information at the top of every subsystem in design.
      mask Display:
      | NxtrConf = 'Nexteer Confidential';
      | 
      | sys = bdroot; %handle for the current model ("system")
      | first = get_param(sys,'Created');
      | first = first(end-3:end);  %year is last four digits
      | 
      | last = get_param(sys,'LastModifiedDate');
      | if isempty(last)
      |     last = datestr(now,'yyyy');
      | else
      |     last = last(end-3:end);
      | end
      | 
      | if strcmp(first,last)
      |     fprintf('%s -- Copyright %s Nexteer',NxtrConf,first)
      | else
      |     fprintf('%s -- %s%s- %s Nexteer',NxtrConf,char(169),first,last)
      | end
  Display4 : Display
  If : If  RequirementInfo={'linktype_rmi_doors' '0000c46e (/ESG Group/FDD Module Requirements/EA4 Specific/ES209A CurrMeasCorrln)' '#ES209A_259' 'true' 'REQ: ES209A_259' '' ; 'linktype_rmi_doors' '0000c46e (/ESG Group/FDD Module Requirements/EA4 Specific/ES209A CurrMeasCorrln)' '#ES209A_261' 'true' 'REQ: ES209A_261' '' } %GIDa_3564d8ec_b0ac_428d_8c97_1e8ed5060a69  NumInputs=2  IfExpression=u1<u2
  If Action Subsystem : Subsystem  RequirementInfo={'linktype_rmi_doors' '0000c46e (/ESG Group/FDD Module Requirements/EA4 Specific/ES209A CurrMeasCorrln)' '#ES209A_261' 'true' 'REQ: ES209A_261' '' } %GIDa_867ed387_085a_4e0f_8637_512c724c9cec  TreatAsAtomicUnit=on
  If Action Subsystem1 : Subsystem  RequirementInfo={'linktype_rmi_doors' '0000c46e (/ESG Group/FDD Module Requirements/EA4 Specific/ES209A CurrMeasCorrln)' '#ES209A_259' 'true' 'REQ: ES209A_259' '' } %GIDa_4eb2a7af_087d_4492_b320_198abaca1be9  TreatAsAtomicUnit=on
  Merge : Merge
  ImdtCorrlnDEF : Outport
  CurrMotSumDEF : Outport  Port=2
  wires:
  If/1 -> If Action Subsystem/Action
  MotCurrCorrdD/1 -> Add/1
  MotCurrCorrdF/1 -> Add/3
  MotCurrCorrdE/1 -> Add/2
  If/2 -> If Action Subsystem1/Action
  If Action Subsystem/1(ImdtCorrlnABC) -> Merge/1
  If Action Subsystem1/1(ImdtCorrlnABC) -> Merge/2
  Merge/1 -> ImdtCorrlnDEF/1
  Constant/1 -> Display4/1, If/2
  Add/1 -> Abs/1
  Abs/1 -> CurrMotSumDEF/1, If/1

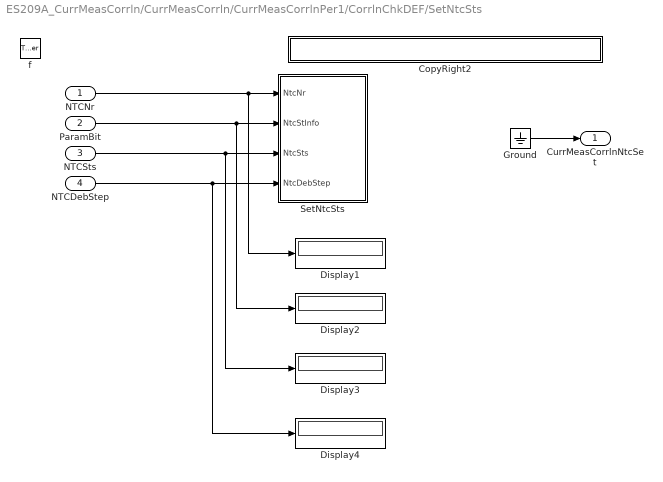
== system ES209A_CurrMeasCorrln/CurrMeasCorrln/CurrMeasCorrlnPer1/CorrlnChkDEF/SetNtcSts ==
  NTCNr : Inport
  ParamBit : Inport  Port=2
  NTCSts : Inport  Port=3
  NTCDebStep : Inport  Port=4
  f : TriggerPort  TriggerType=function-call
      settings: CopyFcn=Stateflow.SLINSF.SimulinkMan.removeBlockPreDeleteFcn  PreDeleteFcn=Stateflow.SLINSF.SimulinkMan.unsafePredeleteFcn
  CopyRight2 : Subsystem  Description=|  mask(Copyright Information){none=on}
      | Copyright info block.                                               
      |                                                                     
      | Place copyright information at the top of every subsystem in design.
      mask prompts: none "No parameters"
      mask help: Place copyright information at the top of every subsystem in design.
      mask Display:
      | NxtrConf = 'Nexteer Confidential';
      | 
      | sys = bdroot; %handle for the current model ("system")
      | first = get_param(sys,'Created');
      | first = first(end-3:end);  %year is last four digits
      | 
      | last = get_param(sys,'LastModifiedDate');
      | if isempty(last)
      |     last = datestr(now,'yyyy');
      | else
      |     last = last(end-3:end);
      | end
      | 
      | if strcmp(first,last)
      |     fprintf('%s -- Copyright %s Nexteer',NxtrConf,first)
      | else
      |     fprintf('%s -- %s%s- %s Nexteer',NxtrConf,char(169),first,last)
      | end
  Display{1..4} (4 alike) : Display
  Ground : Ground
  SetNtcSts : Subsystem  RequirementInfo={} %GIDa_78c0dfd7_f678_47ed_bf3d_29c9c3ca89e9  TreatAsAtomicUnit=on
      settings: RTWSystemCode=Inline
  CurrMeasCorrlnNtcSet : Outport
  wires:
  Ground/1 -> CurrMeasCorrlnNtcSet/1
  NTCDebStep/1 -> Display4/1, SetNtcSts/4(NtcDebStep)
  NTCSts/1 -> Display3/1, SetNtcSts/3(NtcSts)
  ParamBit/1 -> Display2/1, SetNtcSts/2(NtcStInfo)
  NTCNr/1 -> Display1/1, SetNtcSts/1(NtcNr)

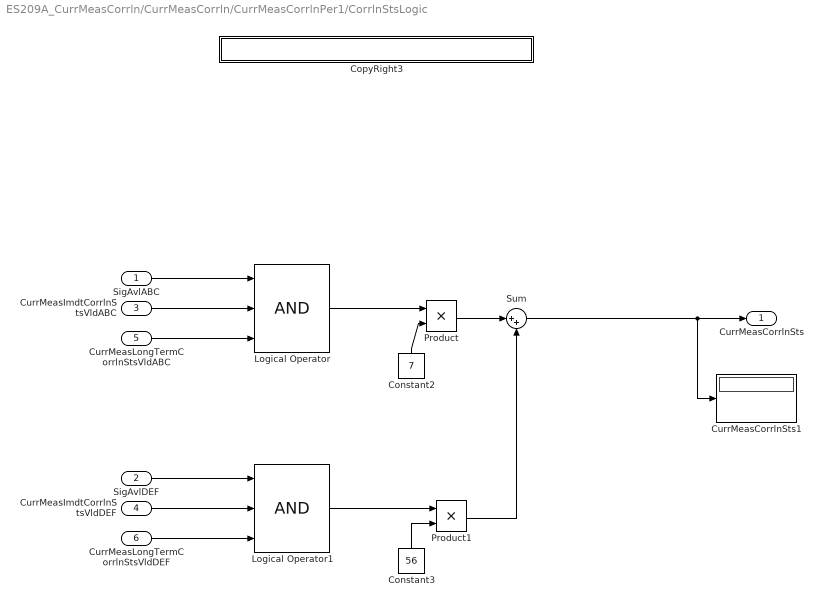
== system ES209A_CurrMeasCorrln/CurrMeasCorrln/CurrMeasCorrlnPer1/CorrlnStsLogic ==
  SigAvlABC : Inport  RequirementInfo={} %GIDa_1f617465_2337_4da1_8acb_1bffe5ca6427
  SigAvlDEF : Inport  RequirementInfo={} %GIDa_c4a2866c_c34d_4776_98a1_c7f906747e7a  Port=2
  CurrMeasImdtCorrlnStsVldABC : Inport  RequirementInfo={} %GIDa_785dc32e_87de_4769_b284_a2b7bce756ce  Port=3
  CurrMeasImdtCorrlnStsVldDEF : Inport  RequirementInfo={} %GIDa_1a7055a1_a3ee_465a_8a5c_191e71c89df9  Port=4
  CurrMeasLongTermCorrlnStsVldABC : Inport  RequirementInfo={} %GIDa_799b4ced_3b86_449c_a738_e296cfc802c2  Port=5
  CurrMeasLongTermCorrlnStsVldDEF : Inport  RequirementInfo={} %GIDa_139f842b_1b8c_4971_9327_4994156f71c1  Port=6
  Constant2 : Constant  RequirementInfo={'linktype_rmi_doors' '0000c46e (/ESG Group/FDD Module Requirements/EA4 Specific/ES209A CurrMeasCorrln)' '#ES209A_211' 'true' 'REQ: ES209A_211' '' } %GIDa_8d5a5ff7_4770_4f90_9fa4_b00de22041dd  Value=7  OutDataTypeStr=uint8
  Constant3 : Constant  RequirementInfo={'linktype_rmi_doors' '0000c46e (/ESG Group/FDD Module Requirements/EA4 Specific/ES209A CurrMeasCorrln)' '#ES209A_222' 'true' 'REQ: ES209A_222' '' } %GIDa_bacdb310_f3a1_41c5_a86b_e6a5bba257c2  Value=56  OutDataTypeStr=uint8
  CopyRight3 : Subsystem  Description=|  mask(Copyright Information){none=on}
      | Copyright info block.                                               
      |                                                                     
      | Place copyright information at the top of every subsystem in design.
      mask prompts: none "No parameters"
      mask help: Place copyright information at the top of every subsystem in design.
      mask Display:
      | NxtrConf = 'Nexteer Confidential';
      | 
      | sys = bdroot; %handle for the current model ("system")
      | first = get_param(sys,'Created');
      | first = first(end-3:end);  %year is last four digits
      | 
      | last = get_param(sys,'LastModifiedDate');
      | if isempty(last)
      |     last = datestr(now,'yyyy');
      | else
      |     last = last(end-3:end);
      | end
      | 
      | if strcmp(first,last)
      |     fprintf('%s -- Copyright %s Nexteer',NxtrConf,first)
      | else
      |     fprintf('%s -- %s%s- %s Nexteer',NxtrConf,char(169),first,last)
      | end
  CurrMeasCorrlnSts1 : Display
  Logical Operator : Logic  RequirementInfo={'linktype_rmi_doors' '0000c46e (/ESG Group/FDD Module Requirements/EA4 Specific/ES209A CurrMeasCorrln)' '#ES209A_211' 'true' 'REQ: ES209A_211' '' } %GIDa_95ac31da_dd15_45d3_b021_fd316b7dab15  Inputs=3  IconShape=distinctive  AllPortsSameDT=off  OutDataTypeStr=boolean
  Logical Operator1 : Logic  RequirementInfo={'linktype_rmi_doors' '0000c46e (/ESG Group/FDD Module Requirements/EA4 Specific/ES209A CurrMeasCorrln)' '#ES209A_222' 'true' 'REQ: ES209A_222' '' } %GIDa_01fff2b3_b0d4_4edb_b5a0_4d16ebef0425  Inputs=3  IconShape=distinctive  AllPortsSameDT=off  OutDataTypeStr=boolean
  Product : Product  RequirementInfo={'linktype_rmi_doors' '0000c46e (/ESG Group/FDD Module Requirements/EA4 Specific/ES209A CurrMeasCorrln)' '#ES209A_211' 'true' 'REQ: ES209A_211' '' } %GIDa_7273919c_7ae7_4540_a15c_07d5a24b73d0
  Product1 : Product  RequirementInfo={'linktype_rmi_doors' '0000c46e (/ESG Group/FDD Module Requirements/EA4 Specific/ES209A CurrMeasCorrln)' '#ES209A_222' 'true' 'REQ: ES209A_222' '' } %GIDa_bc9ce5ec_9225_4253_b211_d2111275c1a7
  Sum : Sum  Inputs=|++
  CurrMeasCorrlnSts : Outport  RequirementInfo={} %GIDa_25dc6e15_0c00_4056_8079_e614d68af1eb
  wires:
  Logical Operator/1 -> Product/1
  Logical Operator1/1 -> Product1/1
  Product/1 -> Sum/1
  Product1/1 -> Sum/2
  Sum/1 -> CurrMeasCorrlnSts1/1, CurrMeasCorrlnSts/1
  Constant2/1 -> Product/2
  Constant3/1 -> Product1/2
  CurrMeasImdtCorrlnStsVldABC/1 -> Logical Operator/2
  SigAvlABC/1 -> Logical Operator/1
  CurrMeasLongTermCorrlnStsVldABC/1 -> Logical Operator/3
  CurrMeasImdtCorrlnStsVldDEF/1 -> Logical Operator1/2
  CurrMeasLongTermCorrlnStsVldDEF/1 -> Logical Operator1/3
  SigAvlDEF/1 -> Logical Operator1/1

== system ES209A_CurrMeasCorrln/CurrMeasCorrln/CurrMeasCorrlnPer1/FltInj_u08 ==
  note: This block requires no modification by FDD author.
      |
      | This block does not actually simulate any fault injection.  It is simply a pass-thru.
      |
      | Input port (#2) simply terminates its signal, but we are trying to force the FDD author
      | to properly use the FltInjectionLocType enumeration in FDD model.
  note: EA4.x Fault Injection
  Sig : Inport
  "LocnKey  " : Inport  Port=2  OutDataTypeStr=uint16
  CopyRight1 : Subsystem  Description=|  mask(Copyright Information){none=on}
      | Copyright info block.                                               
      |                                                                     
      | Place copyright information at the top of every subsystem in design.
      mask prompts: none "No parameters"
      mask help: Place copyright information at the top of every subsystem in design.
      mask Display:
      | NxtrConf = 'Nexteer Confidential';
      | 
      | sys = bdroot; %handle for the current model ("system")
      | first = get_param(sys,'Created');
      | if(isempty(first))
      |     first = datestr(now,'yyyy');
      | else
      |     first = first(end-3:end);  %year is last four digits
      | end
      | 
      | last = get_param(sys,'LastModifiedDate');
      | if isempty(last)
      |     last = datestr(now,'yyyy');
      | else
      |     last = last(end-3:end);
      | end
      | 
      | if strcmp(first,last)
      |     fprintf('%s -- Copyright %s Nexteer',NxtrConf,first)
      | else
      |     fprintf('%s -- %s%s- %s Nexteer',NxtrConf,char(169),first,last)
      | end
  Terminator : Terminator
  Sig_Out : Outport
  wires:
  Sig/1 -> Sig_Out/1
  "LocnKey  "/1 -> Terminator/1
